simulink model "Trigger_Subsystem_And_Func_Call"  (R2016b)
settings: Solver=FixedStepDiscrete  StartTime=0.0  StopTime=10.0  RelTol=1e-3
libraries: simulink x1
settings Model: Creator=Saher Ghanem  LastModifiedBy=Saher Ghanem
settings OptimizationCC: DefaultParameterBehavior=Inlined
settings DebuggingCC: ParameterTunabilityLossMsg=error
settings RTWCC: SystemTargetFile=ert.tlc  GenCodeOnly=on  TemplateMakefile=ert_default_tmf  Description=Embedded Coder  GenerateReport=on  IncludeHyperlinkInReport=on  LaunchReport=on  GenerateTraceInfo=on  GenerateTraceReport=on  GenerateTraceReportSl=on  GenerateTraceReportSf=on  GenerateTraceReportEml=on
settings CodeAppCC: ForceParamTrailComments=on  IgnoreCustomStorageClasses=off  OperatorAnnotations=on  SimulinkDataObjDesc=on  SFDataObjDesc=on  MATLABFcnDesc=on  InsertBlockDesc=on  MATLABSourceComments=on
settings ERTTargetCC: TargetLangStandard=C99 (ISO)  GenerateSampleERTMain=on  InlinedParameterPlacement=NonHierarchical  ERTCustomFileTemplate=example_file_process.tlc  EnableUserReplacementTypes=on

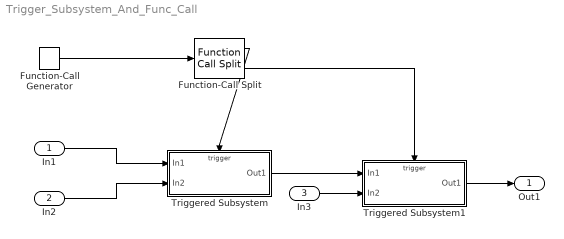
== system Trigger_Subsystem_And_Func_Call ==
  In1 : Inport
  In2 : Inport  Port=2
  In3 : Inport  Port=3
  Function-Call Generator : simulink/Ports & Subsystems/Function-Call Generator  sample_time=1  numberOfIterations=1
  Function-Call Split : FunctionCallSplit  NumOutputPorts=2
  Triggered Subsystem : Subsystem  TreatAsAtomicUnit=on
  Triggered Subsystem1 : Subsystem  TreatAsAtomicUnit=on
  Out1 : Outport
  wires:
  In1/1 -> Triggered Subsystem/1(In1)
  In2/1 -> Triggered Subsystem/2(In2)
  Triggered Subsystem/1(Out1) -> Triggered Subsystem1/1(In1)
  Function-Call Generator/1 -> Function-Call Split/1
  In3/1 -> Triggered Subsystem1/2(In2)
  Function-Call Split/1 -> Triggered Subsystem/Trigger
  Function-Call Split/2 -> Triggered Subsystem1/Trigger
  Triggered Subsystem1/1(Out1) -> Out1/1

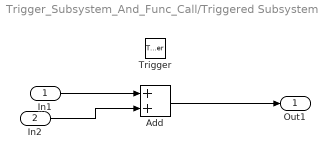
== system Trigger_Subsystem_And_Func_Call/Triggered Subsystem ==
  In1 : Inport
  In2 : Inport  Port=2
  Trigger : TriggerPort  TriggerType=function-call  VariantControl=Variant
  Add : Sum
  Out1 : Outport
  wires:
  In1/1 -> Add/1
  In2/1 -> Add/2
  Add/1 -> Out1/1

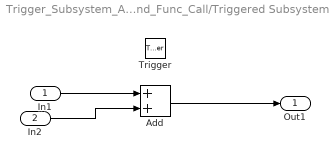
== system Trigger_Subsystem_And_Func_Call/Triggered Subsystem1 ==
  In1 : Inport
  In2 : Inport  Port=2
  Trigger : TriggerPort  TriggerType=function-call  VariantControl=Variant
  Add : Sum
  Out1 : Outport
  wires:
  In1/1 -> Add/1
  In2/1 -> Add/2
  Add/1 -> Out1/1
